simulink model "solar_collector_model_2019b"  (R2019b)
settings: Solver=VariableStepAuto  StartTime=0.0  StopTime=8760  RelTol=1e-3
values from neighbouring files (symbols this model uses):
  a1 = 8*eta/C    (= 0.000491228070175)    [solar_collector.m]
  a2 = -UL_1*Ac/C    (= -0.00290974481659)    [solar_collector.m]
  a3 = -UL_2*Ac/C    (= -7.48006379585e-06)    [solar_collector.m]
  a4 = V^-1    (= 333.333333333)    [solar_collector.m]
  a5 = -a4    (= -333.333333333)    [solar_collector.m]
settings Model: Creator=Mariana  LastModifiedBy=Mariana

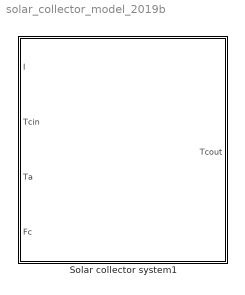
== system solar_collector_model_2019b ==
  Solar collector system1 : Subsystem
      mask Display: image('collector_image.jpg');

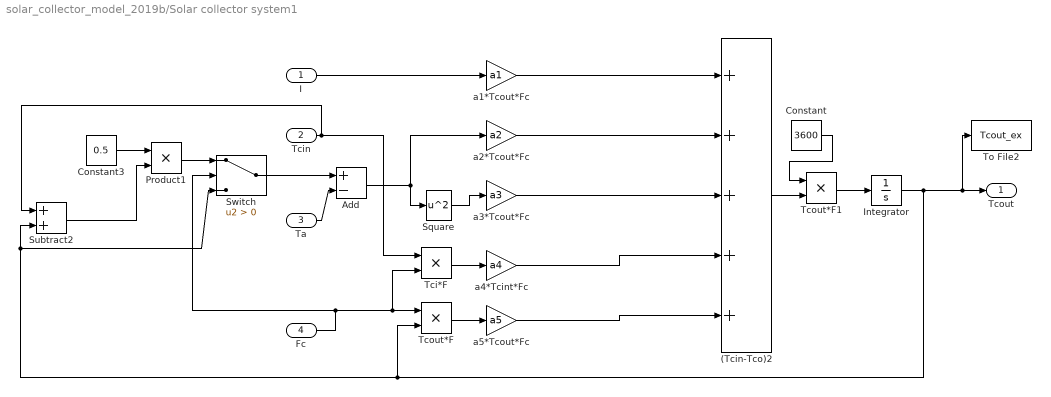
== system solar_collector_model_2019b/Solar collector system1 ==
  I : Inport
  Tcin : Inport  Port=2
  Ta : Inport  Port=3
  Fc : Inport  Port=4
  (Tcin-Tco)2 : Sum  Inputs=+++++
  Add : Sum  Inputs=+-
  Constant : Constant  Value=3600
  Constant3 : Constant  Value=0.5
  Integrator : Integrator  InitialCondition=7.5
  Product1 : Product
  Square : Math  Operator=square  SaturateOnIntegerOverflow=on
  Subtract2 : Sum
  Switch : Switch  Criteria=u2 > Threshold  ZeroCross=off
  Tci*F : Product  Inputs=**
  Tcout*F : Product  Inputs=**
  Tcout*F1 : Product  Inputs=**
  To File2 : ToFile  Filename=Tcout_ex  MatrixName=Tcout_ex  SampleTime=1
  a1*Tcout*Fc : Gain  Gain=a1
  a2*Tcout*Fc : Gain  Gain=a2
  a3*Tcout*Fc : Gain  Gain=a3
  a4*Tcint*Fc : Gain  Gain=a4
  "a5*Tcout*Fc " : Gain  Gain=a5
  Tcout : Outport
  wires:
  a1*Tcout*Fc/1 -> (Tcin-Tco)2/1
  Product1/1 -> Switch/1
  Switch/1 -> Add/1
  Subtract2/1 -> Product1/2
  Integrator/1 -> To File2/1, Tcout/1, Subtract2/2, Switch/3, Tcout*F/2
  Tcout*F1/1 -> Integrator/1
  Constant/1 -> Tcout*F1/1
  (Tcin-Tco)2/1 -> Tcout*F1/2
  Square/1 -> a3*Tcout*Fc/1
  Add/1 -> a2*Tcout*Fc/1, Square/1
  Ta/1 -> Add/2
  I/1 -> a1*Tcout*Fc/1
  "a5*Tcout*Fc "/1 -> (Tcin-Tco)2/5
  Fc/1 -> Switch/2, Tci*F/2, Tcout*F/1
  Tcout*F/1 -> "a5*Tcout*Fc "/1
  a4*Tcint*Fc/1 -> (Tcin-Tco)2/4
  Tci*F/1 -> a4*Tcint*Fc/1
  Tcin/1 -> Subtract2/1, Tci*F/1
  a2*Tcout*Fc/1 -> (Tcin-Tco)2/2
  a3*Tcout*Fc/1 -> (Tcin-Tco)2/3
  Constant3/1 -> Product1/1
